simulink model "BDK_thich_nghi_theo_mo_hinh_chuan"  (R2023a)
settings: Solver=ode4  StartTime=0.0  StopTime=100  FixedStep=0.001  RelTol=1e-3
settings Model: Creator=VINH  LastModifiedBy=VINH

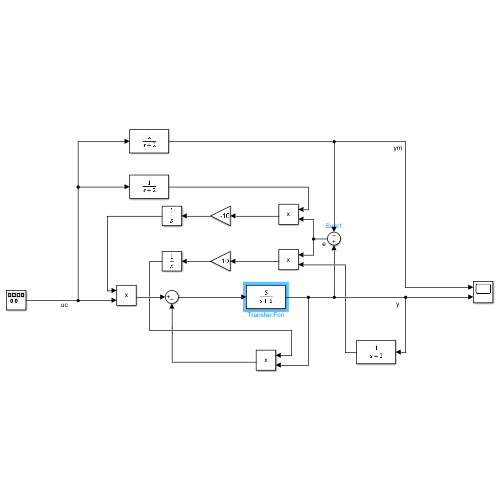
[thumbnail: Simulink's stored preview of the top-level diagram]
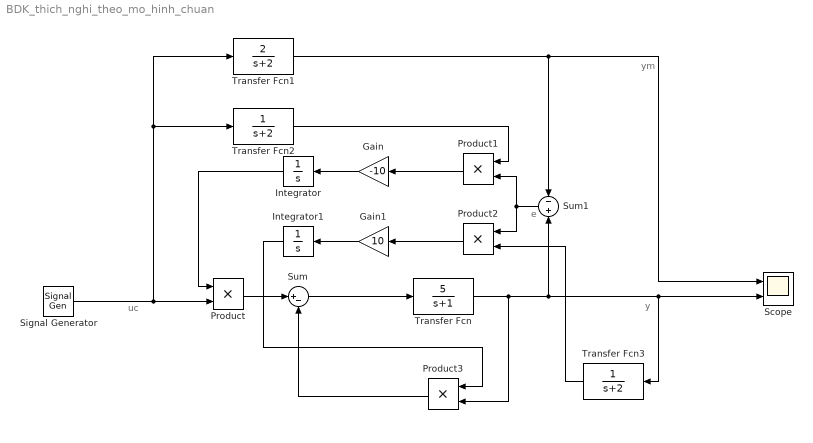
== system BDK_thich_nghi_theo_mo_hinh_chuan ==
  note: uc
  note: e
  note: y
  note: ym
  Gain : Gain  Gain=-10
  Gain1 : Gain  Gain=10
  Integrator : Integrator
  Integrator1 : Integrator
  Product{,1..3} (4 alike) : Product
  Scope : Scope  NumInputPorts=2
  Signal Generator : SignalGenerator  WaveForm=square  Amplitude=0.5  Frequency=0.1
  Sum : Sum  Inputs=|+-
  Sum1 : Sum  Inputs=-|+
  Transfer Fcn : TransferFcn  Numerator=[5]  Denominator=[1 1]
  Transfer Fcn1 : TransferFcn  Numerator=[2]  Denominator=[1 2]
  Transfer Fcn2 : TransferFcn  Denominator=[1 2]
  Transfer Fcn3 : TransferFcn  Denominator=[1 2]
  wires:
  Sum/1 -> Transfer Fcn/1
  Signal Generator/1 -> Transfer Fcn2/1, Transfer Fcn1/1, Product/2
  Transfer Fcn1/1 -> Sum1/1, Scope/1
  Transfer Fcn/1 -> Product3/2, Sum1/2, Transfer Fcn3/1, Scope/2
  Product/1 -> Sum/1
  Transfer Fcn2/1 -> Product1/1
  Sum1/1 -> Product1/2, Product2/1
  Product1/1 -> Gain/1
  Product2/1 -> Gain1/1
  Gain1/1 -> Integrator1/1
  Gain/1 -> Integrator/1
  Integrator/1 -> Product/1
  Integrator1/1 -> Product3/1
  Product3/1 -> Sum/2
  Transfer Fcn3/1 -> Product2/2
